simulink library "csc_hio_hardware_io_mv_lib"  (R2014b)
settings: Solver=ode45  StartTime=0.0  StopTime=10.0  RelTol=1e-3
undefined symbols (not defined in the file or in its folder): fsw_dt
libraries: util_common_lib x3, util_info_lib x1
settings Model: Creator=mstewart  LastModifiedBy=mstewart

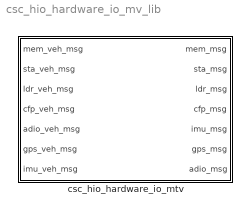
== system csc_hio_hardware_io_mv_lib ==
  csc_hio_hardware_io_mtv : Subsystem  TreatAsAtomicUnit=on  SystemSampleTime=fsw_dt

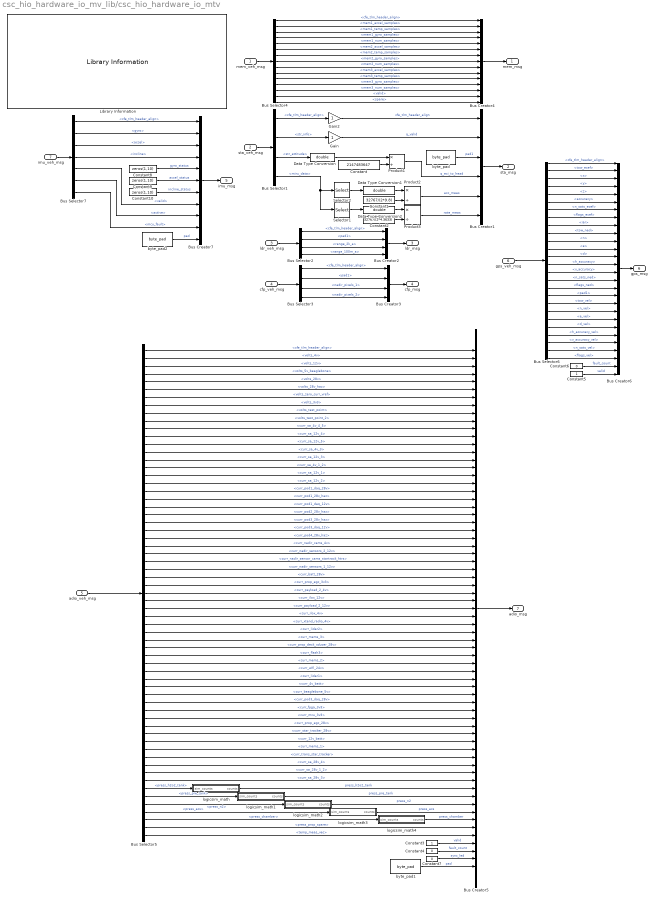
== system csc_hio_hardware_io_mv_lib/csc_hio_hardware_io_mtv ==
  mem_veh_msg : Inport
  sta_veh_msg : Inport  Port=2
  ldr_veh_msg : Inport  Port=3  OutDataTypeStr=Bus: ldr_veh_msg
  cfp_veh_msg : Inport  Port=4  OutDataTypeStr=Bus: cfp_veh_msg
  adio_veh_msg : Inport  Port=5
  gps_veh_msg : Inport  Port=6
  imu_veh_msg : Inport  Port=7
  Bus Creator1 : BusCreator  Inputs=6  OutDataTypeStr=Bus: sta_msg  NonVirtualBus=on
  Bus Creator2 : BusCreator  OutDataTypeStr=Bus: ldr_msg  NonVirtualBus=on
  Bus Creator3 : BusCreator  OutDataTypeStr=Bus: cfp_msg  NonVirtualBus=on
  Bus Creator4 : BusCreator  Inputs=15  OutDataTypeStr=Bus: mem_msg  NonVirtualBus=on
  Bus Creator5 : BusCreator  Inputs=67  OutDataTypeStr=Bus: adio_msg  NonVirtualBus=on
  Bus Creator6 : BusCreator  Inputs=28  OutDataTypeStr=Bus: gps_msg  NonVirtualBus=on
  Bus Creator7 : BusCreator  Inputs=11  OutDataTypeStr=Bus: imu_msg  NonVirtualBus=on
  Bus Selector1 : BusSelector  OutputSignals=fused_attitude.cfe_tlm_header_align,fused_attitude.str_info,fused_attitude.str_attitude,miru_data.miru_data
  Bus Selector2 : BusSelector  OutputSignals=cfe_tlm_header_align,pad1,range_2k_a,range_100m_a
  Bus Selector3 : BusSelector  OutputSignals=cfe_tlm_header_align,pad1,nadir_pixels_1,nadir_pixels_2
  Bus Selector4 : BusSelector  OutputSignals=cfe_tlm_header_align,mem1_accel_samples,mem1_temp_samples,mem1_gyro_samples,mem1_num_samples,mem2_accel_samples,mem2_temp_samples,mem2_gyro_samples,mem2_num_samples,mem3_accel_samples,mem3_temp_samples,mem3_gyro_samples,mem3_num_samples,valid,spare
  Bus Selector5 : BusSelector  OutputSignals=cfe_tlm_header_align,volts_4v,volts_12v,volts_5v_beaglebone,volts_28v,volts_28v_haz,volts_zero_curr_vref,volts_3v3,volts_test_point,volts_test_point_2,curr_sa_4v_4_5,curr_sa_12v_4,curr_sa_12v_5,curr_sa_4v_3,curr_sa_12v_3,curr_sa_4v_1_2,curr_sa_12v_1,curr_sa_12v_2,curr_pod1_daq_28v,curr_pod1_28v_haz,curr_pod1_daq_12v,curr_pod2_28v_haz,curr_pod3_28v_haz,curr_pod3_daq_12v,curr_pod4_28v_haz,curr_nadir_cams_4v,curr_nadir_sensors_2_12v,curr_nadir_sensor_cams_startrack_htrs,curr_nadir_sensors_1_12v,curr_batt_28v,curr_prop_egc_3v3,curr_payload_2_4v,curr_ilox_12v,curr_payload_2_12v,curr_ilox_4v,curr_xtend_radio_4v,curr_lidar2,curr_mems_3,curr_prop_deck_xducer_28v,curr_flash3,curr_mems_2,curr_wifi_24v,curr_lidar1,curr_4v_batt,curr_beaglebone_5v,curr_pod3_daq_28v,curr_fpga_3v3,curr_mcu_3v3,curr_prop_egc_28v,curr_star_tracker_28v,curr_12v_batt,curr_mems_1,curr_trans_star_tracker,curr_sa_28v_4,curr_sa_28v_1_2,curr_sa_28v_3,press_h2o2_tank,press_pre_tank,press_n2,press_acs,press_chamber,press_prop_spare,temp_meas_vec
  Bus Selector6 : BusSelector  OutputSignals=cfe_tlm_header_align,tow_ecef,x,y,z,accuracy,n_sats_ecef,flags_ecef,iar,tow_ned,n,e,d,h_accuracy,v_accuracy,n_sats_ned,flags_ned,pad1,tow_vel,n_vel,e_vel,d_vel,h_accuracy_vel,v_accuracy_vel,n_sats_vel,flags_vel
  Bus Selector7 : BusSelector  OutputSignals=cfe_tlm_header_align,gyro,accel,incline,valid,active,mcu_fault
  Constant : Constant  Value=2147483647  OutDataTypeStr=double
  Constant1 : Constant  Value=32767/(2*9.8)  OutDataTypeStr=double
  Constant10 : Constant  Value=zeros(1,10)  OutDataTypeStr=uint8
  Constant2 : Constant  Value=32767/(2*4.3633)  OutDataTypeStr=double
  Constant3 : Constant  OutDataTypeStr=uint8
  Constant4 : Constant  Value=0  OutDataTypeStr=uint8
  Constant5 : Constant  OutDataTypeStr=uint8
  Constant6 : Constant  Value=0  OutDataTypeStr=uint8
  Constant7 : Constant  Value=0  OutDataTypeStr=uint8
  Constant8 : Constant  Value=zeros(1,10)  OutDataTypeStr=uint8
  Constant9 : Constant  Value=zeros(1,10)  OutDataTypeStr=uint8
  Data Type Conversion : DataTypeConversion  OutDataTypeStr=double
  Data Type Conversion1 : DataTypeConversion  OutDataTypeStr=double
  Data Type Conversion2 : DataTypeConversion  OutDataTypeStr=double
  Gain : Gain  OutDataTypeStr=uint8
  Gain2 : Gain  OutDataTypeStr=uint8
  Library Information : util_info_lib/Library Information  owner='NONE'
  Product1 : Product  Inputs=*/  RndMeth=Zero
  Product2 : Product  Inputs=*/  RndMeth=Zero
  Product3 : Product  Inputs=*/  RndMeth=Zero
  Selector1 : Selector  NumberOfDimensions=2  InputPortWidth=11  IndexOptions=Select all,Index vector (dialog)  Indices=1,[9 10 11]  OutputSizes=1,1
  Selector2 : Selector  NumberOfDimensions=2  InputPortWidth=11  IndexOptions=Select all,Index vector (dialog)  Indices=1,[1:8]  OutputSizes=1,1
  byte_pad : util_common_lib/byte_pad  n_bytes=3
  byte_pad1 : util_common_lib/byte_pad  n_bytes=1
  byte_pad2 : util_common_lib/byte_pad  n_bytes=2
  logicsim_math : Subsystem
  logicsim_math1 : Subsystem
  logicsim_math2 : Subsystem
  logicsim_math3 : Subsystem
  logicsim_math4 : Subsystem
  mem_msg : Outport  OutDataTypeStr=Bus: mem_msg
  sta_msg : Outport  Port=2  OutDataTypeStr=Bus: sta_msg
  ldr_msg : Outport  Port=3  OutDataTypeStr=Bus: ldr_msg
  cfp_msg : Outport  Port=4  OutDataTypeStr=Bus: cfp_msg
  imu_msg : Outport  Port=5  OutDataTypeStr=Bus: imu_msg
  gps_msg : Outport  Port=6
  adio_msg : Outport  Port=7  OutDataTypeStr=Bus: adio_msg
  wires:
  Constant10/1 -> Bus Creator7/7  "incline_status"
  Constant9/1 -> Bus Creator7/6  "accel_status"
  Constant8/1 -> Bus Creator7/5  "gyro_status"
  byte_pad2/1 -> Bus Creator7/11  "pad"
  byte_pad1/1 -> Bus Creator5/67  "pad"
  Constant7/1 -> Bus Creator5/66  "sync_led"
  logicsim_math4/1(counts) -> Bus Creator5/61  "press_chamber"
  logicsim_math3/1(counts) -> Bus Creator5/60  "press_acs"
  logicsim_math2/1(counts) -> Bus Creator5/59  "press_n2"
  logicsim_math1/1(counts) -> Bus Creator5/58  "press_pre_tank"
  logicsim_math/1(counts) -> Bus Creator5/57  "press_h2o2_tank"
  Bus Creator5/1 -> adio_msg/1
  Bus Selector5/63 -> Bus Creator5/63  "<temp_meas_vec>"
  Bus Selector5/62 -> Bus Creator5/62  "<press_prop_spare>"
  Bus Selector5/61 -> logicsim_math4/1(sim_counts)  "<press_chamber>"
  Bus Selector5/60 -> logicsim_math3/1(sim_counts)  "<press_acs>"
  Bus Selector5/59 -> logicsim_math2/1(sim_counts)  "<press_n2>"
  Bus Selector5/58 -> logicsim_math1/1(sim_counts)  "<press_pre_tank>"
  Bus Selector5/57 -> logicsim_math/1(sim_counts)  "<press_h2o2_tank>"
  Bus Selector5/56 -> Bus Creator5/56  "<curr_sa_28v_3>"
  Bus Selector5/55 -> Bus Creator5/55  "<curr_sa_28v_1_2>"
  Bus Selector5/54 -> Bus Creator5/54  "<curr_sa_28v_4>"
  Bus Selector5/53 -> Bus Creator5/53  "<curr_trans_star_tracker>"
  Bus Selector5/52 -> Bus Creator5/52  "<curr_mems_1>"
  Bus Selector5/51 -> Bus Creator5/51  "<curr_12v_batt>"
  Bus Selector5/50 -> Bus Creator5/50  "<curr_star_tracker_28v>"
  Bus Selector5/49 -> Bus Creator5/49  "<curr_prop_egc_28v>"
  Bus Selector5/48 -> Bus Creator5/48  "<curr_mcu_3v3>"
  Bus Selector5/47 -> Bus Creator5/47  "<curr_fpga_3v3>"
  Bus Selector5/46 -> Bus Creator5/46  "<curr_pod3_daq_28v>"
  Bus Selector5/45 -> Bus Creator5/45  "<curr_beaglebone_5v>"
  Bus Selector5/44 -> Bus Creator5/44  "<curr_4v_batt>"
  Bus Selector5/43 -> Bus Creator5/43  "<curr_lidar1>"
  Bus Selector5/42 -> Bus Creator5/42  "<curr_wifi_24v>"
  Bus Selector5/41 -> Bus Creator5/41  "<curr_mems_2>"
  Bus Selector5/40 -> Bus Creator5/40  "<curr_flash3>"
  Bus Selector5/39 -> Bus Creator5/39  "<curr_prop_deck_xducer_28v>"
  Bus Selector5/38 -> Bus Creator5/38  "<curr_mems_3>"
  Bus Selector5/37 -> Bus Creator5/37  "<curr_lidar2>"
  Bus Selector5/36 -> Bus Creator5/36  "<curr_xtend_radio_4v>"
  Bus Selector5/35 -> Bus Creator5/35  "<curr_ilox_4v>"
  Bus Selector5/34 -> Bus Creator5/34  "<curr_payload_2_12v>"
  Bus Selector5/33 -> Bus Creator5/33  "<curr_ilox_12v>"
  Bus Selector5/32 -> Bus Creator5/32  "<curr_payload_2_4v>"
  Bus Selector5/31 -> Bus Creator5/31  "<curr_prop_egc_3v3>"
  Bus Selector5/30 -> Bus Creator5/30  "<curr_batt_28v>"
  Bus Selector5/29 -> Bus Creator5/29  "<curr_nadir_sensors_1_12v>"
  Bus Selector5/28 -> Bus Creator5/28  "<curr_nadir_sensor_cams_startrack_htrs>"
  Bus Selector5/27 -> Bus Creator5/27  "<curr_nadir_sensors_2_12v>"
  Bus Selector5/26 -> Bus Creator5/26  "<curr_nadir_cams_4v>"
  Bus Selector5/25 -> Bus Creator5/25  "<curr_pod4_28v_haz>"
  Bus Selector5/24 -> Bus Creator5/24  "<curr_pod3_daq_12v>"
  Bus Selector5/23 -> Bus Creator5/23  "<curr_pod3_28v_haz>"
  Bus Selector5/22 -> Bus Creator5/22  "<curr_pod2_28v_haz>"
  Bus Selector5/21 -> Bus Creator5/21  "<curr_pod1_daq_12v>"
  Bus Selector5/20 -> Bus Creator5/20  "<curr_pod1_28v_haz>"
  Bus Selector5/19 -> Bus Creator5/19  "<curr_pod1_daq_28v>"
  Bus Selector5/18 -> Bus Creator5/18  "<curr_sa_12v_2>"
  Bus Selector5/17 -> Bus Creator5/17  "<curr_sa_12v_1>"
  Bus Selector5/16 -> Bus Creator5/16  "<curr_sa_4v_1_2>"
  Bus Selector5/15 -> Bus Creator5/15  "<curr_sa_12v_3>"
  Bus Selector5/14 -> Bus Creator5/14  "<curr_sa_4v_3>"
  Bus Selector5/13 -> Bus Creator5/13  "<curr_sa_12v_5>"
  Bus Selector5/12 -> Bus Creator5/12  "<curr_sa_12v_4>"
  Bus Selector5/11 -> Bus Creator5/11  "<curr_sa_4v_4_5>"
  Bus Selector5/10 -> Bus Creator5/10  "<volts_test_point_2>"
  Bus Selector5/9 -> Bus Creator5/9  "<volts_test_point>"
  Bus Selector5/8 -> Bus Creator5/8  "<volts_3v3>"
  Bus Selector5/7 -> Bus Creator5/7  "<volts_zero_curr_vref>"
  Bus Selector5/6 -> Bus Creator5/6  "<volts_28v_haz>"
  Bus Selector5/5 -> Bus Creator5/5  "<volts_28v>"
  Bus Selector5/4 -> Bus Creator5/4  "<volts_5v_beaglebone>"
  Bus Selector5/3 -> Bus Creator5/3  "<volts_12v>"
  Bus Selector5/2 -> Bus Creator5/2  "<volts_4v>"
  Bus Selector5/1 -> Bus Creator5/1  "<cfe_tlm_header_align>"
  Bus Selector6/26 -> Bus Creator6/26  "<flags_vel>"
  Bus Selector6/25 -> Bus Creator6/25  "<n_sats_vel>"
  Bus Selector6/24 -> Bus Creator6/24  "<v_accuracy_vel>"
  Bus Selector6/23 -> Bus Creator6/23  "<h_accuracy_vel>"
  Bus Selector6/22 -> Bus Creator6/22  "<d_vel>"
  Bus Selector6/21 -> Bus Creator6/21  "<e_vel>"
  Bus Selector6/20 -> Bus Creator6/20  "<n_vel>"
  Bus Selector6/19 -> Bus Creator6/19  "<tow_vel>"
  Bus Selector6/18 -> Bus Creator6/18  "<pad1>"
  Bus Selector7/7 -> Bus Creator7/10  "<mcu_fault>"
  Bus Selector7/6 -> Bus Creator7/9  "<active>"
  Bus Selector7/5 -> Bus Creator7/8  "<valid>"
  Bus Selector7/4 -> Bus Creator7/4  "<incline>"
  Bus Selector7/3 -> Bus Creator7/3  "<accel>"
  Bus Selector7/2 -> Bus Creator7/2  "<gyro>"
  Bus Selector7/1 -> Bus Creator7/1  "<cfe_tlm_header_align>"
  Bus Creator7/1 -> imu_msg/1
  imu_veh_msg/1 -> Bus Selector7/1
  Constant5/1 -> Bus Creator6/28  "valid"
  Constant6/1 -> Bus Creator6/27  "fault_count"
  Bus Selector6/1 -> Bus Creator6/1  "<cfe_tlm_header_align>"
  Bus Selector6/2 -> Bus Creator6/2  "<tow_ecef>"
  Bus Selector6/3 -> Bus Creator6/3  "<x>"
  Bus Selector6/17 -> Bus Creator6/17  "<flags_ned>"
  Bus Selector6/4 -> Bus Creator6/4  "<y>"
  Bus Selector6/16 -> Bus Creator6/16  "<n_sats_ned>"
  Bus Selector6/15 -> Bus Creator6/15  "<v_accuracy>"
  Bus Selector6/5 -> Bus Creator6/5  "<z>"
  Bus Selector6/14 -> Bus Creator6/14  "<h_accuracy>"
  Bus Selector6/6 -> Bus Creator6/6  "<accuracy>"
  Bus Selector6/7 -> Bus Creator6/7  "<n_sats_ecef>"
  Bus Selector6/13 -> Bus Creator6/13  "<d>"
  Bus Selector6/8 -> Bus Creator6/8  "<flags_ecef>"
  Bus Selector6/12 -> Bus Creator6/12  "<e>"
  Bus Selector6/11 -> Bus Creator6/11  "<n>"
  Bus Selector6/9 -> Bus Creator6/9  "<iar>"
  Bus Selector6/10 -> Bus Creator6/10  "<tow_ned>"
  Bus Creator6/1 -> gps_msg/1
  gps_veh_msg/1 -> Bus Selector6/1
  Constant3/1 -> Bus Creator5/64  "valid"
  Constant4/1 -> Bus Creator5/65  "fault_count"
  adio_veh_msg/1 -> Bus Selector5/1
  Bus Selector4/15 -> Bus Creator4/15  "<spare>"
  Bus Selector4/14 -> Bus Creator4/14  "<valid>"
  Bus Selector4/13 -> Bus Creator4/13  "<mem3_num_samples>"
  Bus Selector4/9 -> Bus Creator4/9  "<mem2_num_samples>"
  Bus Selector4/5 -> Bus Creator4/5  "<mem1_num_samples>"
  Bus Selector4/12 -> Bus Creator4/12  "<mem3_gyro_samples>"
  Bus Selector4/11 -> Bus Creator4/11  "<mem3_temp_samples>"
  Bus Selector4/10 -> Bus Creator4/10  "<mem3_accel_samples>"
  Bus Creator4/1 -> mem_msg/1
  Bus Selector4/1 -> Bus Creator4/1  "<cfe_tlm_header_align>"
  Bus Selector4/2 -> Bus Creator4/2  "<mem1_accel_samples>"
  Bus Selector4/3 -> Bus Creator4/3  "<mem1_temp_samples>"
  Bus Selector4/4 -> Bus Creator4/4  "<mem1_gyro_samples>"
  Bus Selector4/6 -> Bus Creator4/6  "<mem2_accel_samples>"
  Bus Selector4/8 -> Bus Creator4/8  "<mem2_gyro_samples>"
  Bus Selector4/7 -> Bus Creator4/7  "<mem2_temp_samples>"
  mem_veh_msg/1 -> Bus Selector4/1
  Selector1/1 -> Data Type Conversion2/1
  Data Type Conversion2/1 -> Product3/1
  Constant2/1 -> Product3/2
  Selector2/1 -> Data Type Conversion1/1
  Data Type Conversion1/1 -> Product2/1
  Constant1/1 -> Product2/2
  Data Type Conversion/1 -> Product1/1
  Constant/1 -> Product1/2
  Gain2/1 -> Bus Creator1/1  "cfe_tlm_header_align"
  Product2/1 -> Bus Creator1/5  "acc_meas"
  Bus Selector1/4 -> Selector2/1, Selector1/1  "<miru_data>"
  Product1/1 -> Bus Creator1/4  "q_eci_to_head"
  Gain/1 -> Bus Creator1/2  "q_valid"
  Bus Selector3/1 -> Bus Creator3/1  "<cfe_tlm_header_align>"
  Bus Selector2/1 -> Bus Creator2/1  "<cfe_tlm_header_align>"
  Bus Selector1/1 -> Gain2/1  "<cfe_tlm_header_align>"
  byte_pad/1 -> Bus Creator1/3  "pad1"
  Bus Selector3/4 -> Bus Creator3/4  "<nadir_pixels_2>"
  Bus Selector3/3 -> Bus Creator3/3  "<nadir_pixels_1>"
  Bus Selector3/2 -> Bus Creator3/2  "<pad1>"
  Bus Selector2/4 -> Bus Creator2/4  "<range_100m_a>"
  Bus Selector2/3 -> Bus Creator2/3  "<range_2k_a>"
  Bus Selector2/2 -> Bus Creator2/2  "<pad1>"
  Product3/1 -> Bus Creator1/6  "rate_meas"
  Bus Selector1/3 -> Data Type Conversion/1  "<str_attitude>"
  Bus Selector1/2 -> Gain/1  "<str_info>"
  Bus Creator1/1 -> sta_msg/1
  Bus Creator2/1 -> ldr_msg/1
  Bus Creator3/1 -> cfp_msg/1
  cfp_veh_msg/1 -> Bus Selector3/1
  ldr_veh_msg/1 -> Bus Selector2/1
  sta_veh_msg/1 -> Bus Selector1/1

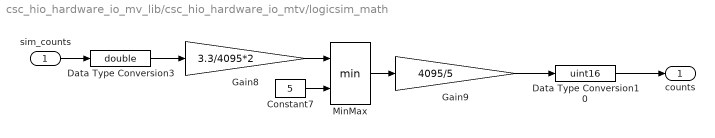
== system csc_hio_hardware_io_mv_lib/csc_hio_hardware_io_mtv/logicsim_math ==
  sim_counts : Inport
  Constant7 : Constant  Value=5  OutDataTypeStr=double
  Data Type Conversion10 : DataTypeConversion  OutDataTypeStr=uint16
  Data Type Conversion3 : DataTypeConversion  OutDataTypeStr=double
  Gain8 : Gain  Gain=3.3/4095*2  OutDataTypeStr=double
  Gain9 : Gain  Gain=4095/5  OutDataTypeStr=double
  MinMax : MinMax  Inputs=2
  counts : Outport
  wires:
  Data Type Conversion10/1 -> counts/1
  Data Type Conversion3/1 -> Gain8/1
  Gain8/1 -> MinMax/1
  sim_counts/1 -> Data Type Conversion3/1
  Gain9/1 -> Data Type Conversion10/1
  MinMax/1 -> Gain9/1
  Constant7/1 -> MinMax/2

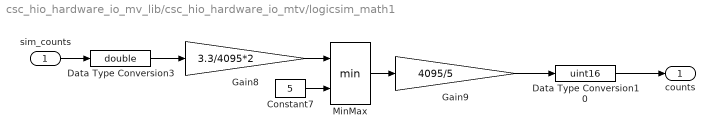
== system csc_hio_hardware_io_mv_lib/csc_hio_hardware_io_mtv/logicsim_math1 ==
  sim_counts : Inport
  Constant7 : Constant  Value=5  OutDataTypeStr=double
  Data Type Conversion10 : DataTypeConversion  OutDataTypeStr=uint16
  Data Type Conversion3 : DataTypeConversion  OutDataTypeStr=double
  Gain8 : Gain  Gain=3.3/4095*2  OutDataTypeStr=double
  Gain9 : Gain  Gain=4095/5  OutDataTypeStr=double
  MinMax : MinMax  Inputs=2
  counts : Outport
  wires:
  Data Type Conversion10/1 -> counts/1
  Data Type Conversion3/1 -> Gain8/1
  Gain8/1 -> MinMax/1
  sim_counts/1 -> Data Type Conversion3/1
  Gain9/1 -> Data Type Conversion10/1
  MinMax/1 -> Gain9/1
  Constant7/1 -> MinMax/2

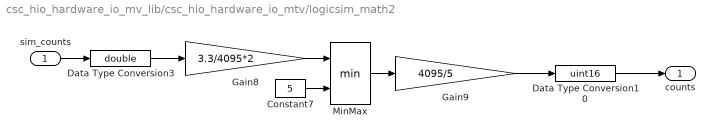
== system csc_hio_hardware_io_mv_lib/csc_hio_hardware_io_mtv/logicsim_math2 ==
  sim_counts : Inport
  Constant7 : Constant  Value=5  OutDataTypeStr=double
  Data Type Conversion10 : DataTypeConversion  OutDataTypeStr=uint16
  Data Type Conversion3 : DataTypeConversion  OutDataTypeStr=double
  Gain8 : Gain  Gain=3.3/4095*2  OutDataTypeStr=double
  Gain9 : Gain  Gain=4095/5  OutDataTypeStr=double
  MinMax : MinMax  Inputs=2
  counts : Outport
  wires:
  Data Type Conversion10/1 -> counts/1
  Data Type Conversion3/1 -> Gain8/1
  Gain8/1 -> MinMax/1
  sim_counts/1 -> Data Type Conversion3/1
  Gain9/1 -> Data Type Conversion10/1
  MinMax/1 -> Gain9/1
  Constant7/1 -> MinMax/2

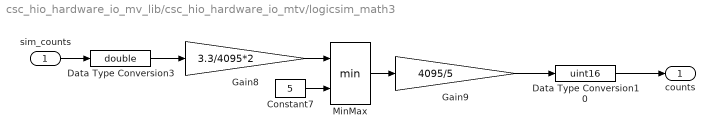
== system csc_hio_hardware_io_mv_lib/csc_hio_hardware_io_mtv/logicsim_math3 ==
  sim_counts : Inport
  Constant7 : Constant  Value=5  OutDataTypeStr=double
  Data Type Conversion10 : DataTypeConversion  OutDataTypeStr=uint16
  Data Type Conversion3 : DataTypeConversion  OutDataTypeStr=double
  Gain8 : Gain  Gain=3.3/4095*2  OutDataTypeStr=double
  Gain9 : Gain  Gain=4095/5  OutDataTypeStr=double
  MinMax : MinMax  Inputs=2
  counts : Outport
  wires:
  Data Type Conversion10/1 -> counts/1
  Data Type Conversion3/1 -> Gain8/1
  Gain8/1 -> MinMax/1
  sim_counts/1 -> Data Type Conversion3/1
  Gain9/1 -> Data Type Conversion10/1
  MinMax/1 -> Gain9/1
  Constant7/1 -> MinMax/2

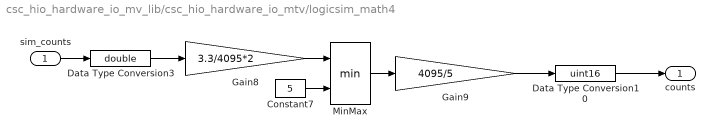
== system csc_hio_hardware_io_mv_lib/csc_hio_hardware_io_mtv/logicsim_math4 ==
  sim_counts : Inport
  Constant7 : Constant  Value=5  OutDataTypeStr=double
  Data Type Conversion10 : DataTypeConversion  OutDataTypeStr=uint16
  Data Type Conversion3 : DataTypeConversion  OutDataTypeStr=double
  Gain8 : Gain  Gain=3.3/4095*2  OutDataTypeStr=double
  Gain9 : Gain  Gain=4095/5  OutDataTypeStr=double
  MinMax : MinMax  Inputs=2
  counts : Outport
  wires:
  Data Type Conversion10/1 -> counts/1
  Data Type Conversion3/1 -> Gain8/1
  Gain8/1 -> MinMax/1
  sim_counts/1 -> Data Type Conversion3/1
  Gain9/1 -> Data Type Conversion10/1
  MinMax/1 -> Gain9/1
  Constant7/1 -> MinMax/2
